simulink model "Circuit1"  (R2018b)
settings: Solver=ode4  StartTime=0.0  StopTime=5  FixedStep=1e-4  RelTol=1e-3
values from neighbouring files (symbols this model uses):
  Be = 1300e6    (= 1300000000)    [Circuit1_load.m]    (also in Circuit2_values.m)
  Cd = 0.7    [Circuit1_load.m]    (also in Circuit2_values.m)
  Dorifice = 2e-2    (= 0.02)    [Circuit1_load.m]    (also in Circuit2_values.m = 0.004)
  Kp = (1.e-3)/(10e5)    (= 1e-09)    [Circuit1_load.m]    (also in Circuit2_values.m; Circut3_values.m)
  pref = 180e5    (= 18000000)    [Circuit1_load.m]    (also in Circuit2_values.m; Circut3_values.m = 17000000)
  rho = 860    [Circuit1_load.m]    (also in Circuit2_values.m; Circut3_values.m)
  tau = 60e-3    (= 0.06)    [Circuit1_load.m]    (also in Circuit2_values.m = 0.03)
  V = 3e-3    (= 0.003)    [Circuit1_load.m]    (also in Circuit2_values.m)
settings Model: Creator=Janne  LastModifiedBy=Janne

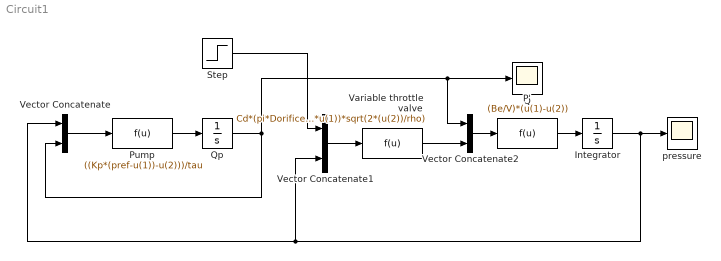
== system Circuit1 ==
  Integrator : Integrator
  P' : Fcn  Expr=(Be/V)*(u(1)-u(2))
  Pump : Fcn  Expr=((Kp*(pref-u(1))-u(2)))/tau
  Q : Scope
  Qp : Integrator
  Step : Step  Time=2  Before=1  After=4  SampleTime=0
  Variable throttle valve : Fcn  Expr=Cd*(pi*Dorifice*u(1))*sqrt(2*(u(2))/rho)
  Vector Concatenate : Concatenate
  Vector Concatenate1 : Concatenate
  Vector Concatenate2 : Concatenate
  pressure : Scope
  wires:
  Pump/1 -> Qp/1
  Qp/1 -> Vector Concatenate2/1, Q/1, Vector Concatenate/2
  Vector Concatenate/1 -> Pump/1
  Vector Concatenate1/1 -> Variable throttle valve/1
  Step/1 -> Vector Concatenate1/1
  Vector Concatenate2/1 -> P'/1
  Variable throttle valve/1 -> Vector Concatenate2/2
  P'/1 -> Integrator/1
  Integrator/1 -> Vector Concatenate/1, Vector Concatenate1/2, pressure/1
